simulink model "simulink_1_zadatak"  (R2013a)
settings: Solver=ode45  StartTime=0.0  StopTime=10.0  RelTol=1e-3
libraries: dspvision x1, dspsnks4 x1
settings Model: SimulationMode=accelerator  Creator=Petra  LastModifiedBy=Petra

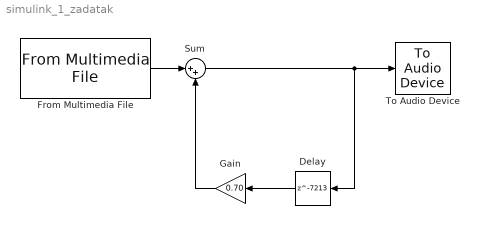
== system simulink_1_zadatak ==
  Delay : Delay  DelayLength=7213  InputProcessing=Columns as channels (frame based)
  From Multimedia File : dspvision/From Multimedia File  inputFilename=C:\Petra\FER\Obrada Informacija\1. Laboratorijska vjezba\0036449369_z3.2-1_a0.70_D7213.wav  loop=on  numPlays=inf  outputStreams=Audio only  videoDataType=single  audioDataType=double  inheritSampleTime=off  userDefinedSampleTime=1/30  noAudioOutput=off  isIntensityVideo=off  fourcc=RGB  colorVideoFormat=Separate color signals  outputEOF=off  dataOrg=Column-major  audioFrameSize=1024  computeAudioFrameSize=off  outSamplingMode=Frame based
  Gain : Gain  Gain=0.70
  Sum : Sum  Inputs=|++
  To Audio Device : dspsnks4/To Audio Device  deviceName=Default  inheritSampleRate=on  sampleRate=44100  deviceDatatype=Determine from input data type  autoBufferSize=on  bufferSize=4096  queueDuration=1.0
  wires:
  Delay/1 -> Gain/1
  From Multimedia File/1 -> Sum/1
  Gain/1 -> Sum/2
  Sum/1 -> Delay/1, To Audio Device/1
